simulink model "test"  (Simulink 8.8)
settings: Solver=ode5  StartTime=0.0  StopTime=inf  FixedStep=0.01  RelTol=1e-3  EnableMultiTasking=on
libraries: WBToolboxLibrary x7
settings Model: SuppressorTable=22 serialization::archive 11 0 3 0 0 0 11 0  Creator=yeshi  LastModifiedBy=yeshi
settings DataIOCC: LimitDataPoints=off  SaveFormat=Dataset  SignalLoggingSaveFormat=Dataset
settings DebuggingCC: UnderspecifiedInitializationDetection=Simplified  MergeDetectMultiDrivingBlocksExec=error  FcnCallInpInsideContextMsg=error  StateNameClashWarn=none
settings HardwareCC: ProdBitPerPointer=64  ProdBitPerSizeT=64  ProdBitPerPtrDiffT=64  ProdLargestAtomicFloat=Float  ProdIntDivRoundTo=Zero  ProdEndianess=LittleEndian  ProdWordSize=64  ProdHWDeviceType=Intel->x86-64 (Windows64)
settings ModelReferenceCC: PropagateSignalLabelsOutOfModel=on
settings GRTTargetCC: CombineOutputUpdateFcns=on  GRTInterface=off

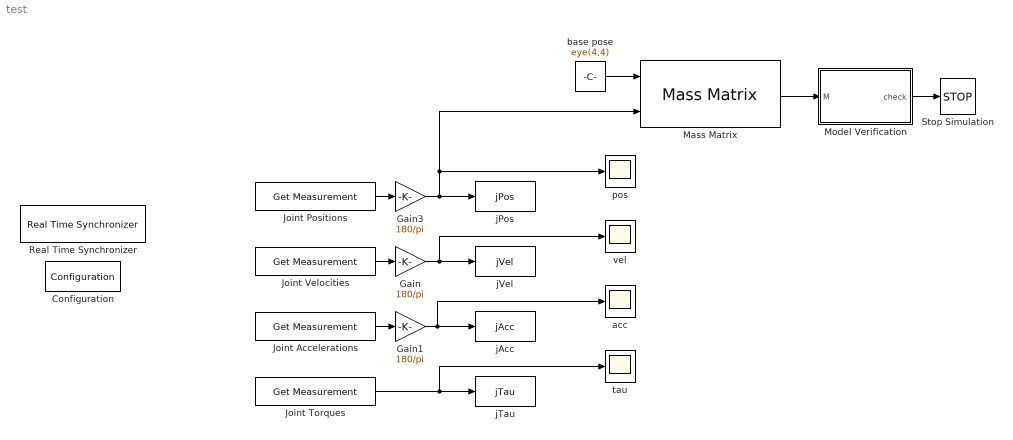
== system test ==
  Configuration : WBToolboxLibrary/Utilities/Configuration  ConfigSource=Workspace  ConfigObject="'HUMAN.WBTConfigRobot   '"
  Gain : Gain  Gain=180/pi
  Gain1 : Gain  Gain=180/pi
  Gain3 : Gain  Gain=180/pi
  Joint Accelerations : WBToolboxLibrary/wholeBodyStates/Get Measurement  measuredType=Joints Acceleration
  Joint Positions : WBToolboxLibrary/wholeBodyStates/Get Measurement  measuredType=Joints Position
  Joint Torques : WBToolboxLibrary/wholeBodyStates/Get Measurement  measuredType=Joints Torque
  Joint Velocities : WBToolboxLibrary/wholeBodyStates/Get Measurement  measuredType=Joints Velocity
  Mass Matrix : WBToolboxLibrary/wholeBodyModel/Dynamics/Mass Matrix
  Model Verification : MATLAB Function  TreatAsAtomicUnit=on
  Real Time Synchronizer : WBToolboxLibrary/Utilities/Real Time Synchronizer  period=0.01
  Stop Simulation : Stop
  acc : Scope
  base pose : Constant  Value=eye(4,4)
  jAcc : ToWorkspace  VariableName=jAcc  SaveFormat=Timeseries  SampleTime=-1
  jPos : ToWorkspace  VariableName=jPos  SaveFormat=Timeseries  SampleTime=-1
  jTau : ToWorkspace  VariableName=jTau  SaveFormat=Timeseries  SampleTime=-1
  jVel : ToWorkspace  VariableName=jVel  SaveFormat=Timeseries  SampleTime=-1
  pos : Scope
  tau : Scope
  vel : Scope
  wires:
  Joint Positions/1 -> Gain3/1
  Joint Velocities/1 -> Gain/1
  Joint Torques/1 -> tau/1, jTau/1
  base pose/1 -> Mass Matrix/1
  Mass Matrix/1 -> Model Verification/1(M)
  Model Verification/1(check) -> Stop Simulation/1
  Gain3/1 -> pos/1, Mass Matrix/2, jPos/1
  Gain/1 -> vel/1, jVel/1
  Joint Accelerations/1 -> Gain1/1
  Gain1/1 -> acc/1, jAcc/1

== matlab function Model Verification ==
  data: M input double; check output double
function check  = verifyModel(M)

    check = 0;
    val = 0;
    %% Mass matrix is symmetric and positive definite
    [s,v,d] = svd(M);
    
    if(min(v(:)) < 0)
        check = 1;
        fprintf('Human model verification failed \n');
    end
    
end
